simulink model "RateAdaptive"  (R2020a)
settings: Solver=FixedStepAuto  StartTime=0.0  StopTime=10.0  FixedStep=1e-3  RelTol=1e-3  EnableMultiTasking=on
settings Model: ExtModeTrigDuration=5  Creator=WinnieTrandinh  LastModifiedBy=WinnieTrandinh
settings OptimizationCC: EnhancedBackFolding=on  PassReuseOutputArgsAs=Individual arguments  ZeroExternalMemoryAtStartup=off  ZeroInternalMemoryAtStartup=off  MaxStackSize=64  OptimizeBlockOrder=speed  DifferentSizesBufferReuse=on  OptimizationCustomize=off  EfficientTunableParamExpr=on
settings DebuggingCC: ParameterTunabilityLossMsg=error
settings HardwareCC: ProdBitPerPointer=32  ProdBitPerSizeT=32  ProdBitPerPtrDiffT=32  ProdLargestAtomicInteger=Long  ProdLargestAtomicFloat=Double  ProdWordSize=32  ProdHWDeviceType=ARM Compatible->ARM Cortex
settings SFSimCC: MATLABDynamicMemAlloc=off
settings RTWCC: SystemTargetFile=ert.tlc  HardwareBoard=NXP FRDM-K64F  TemplateMakefile=ert_default_tmf  Toolchain=GNU Tools for ARM Embedded Processors
settings CodeAppCC: ForceParamTrailComments=on  IgnoreCustomStorageClasses=off  OperatorAnnotations=on  SimulinkDataObjDesc=on  SFDataObjDesc=on  InsertBlockDesc=on

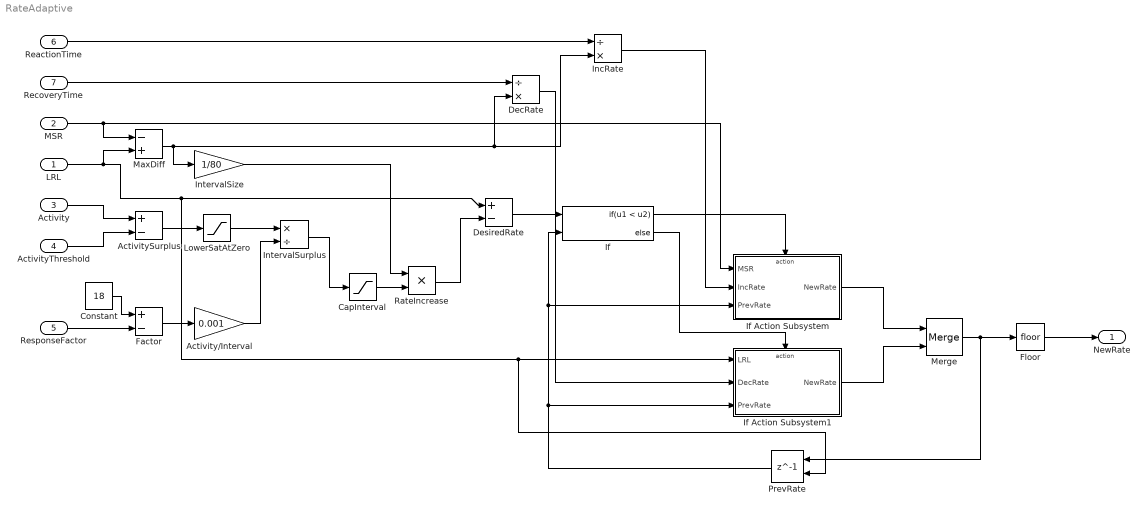
== system RateAdaptive ==
  LRL : Inport  Unit=ms
  MSR : Inport  Port=2  Unit=ms
  Activity : Inport  Port=3
  ActivityThreshold : Inport  Port=4
  ResponseFactor : Inport  Port=5
  ReactionTime : Inport  Port=6  Unit=ms
  RecoveryTime : Inport  Port=7  Unit=ms
  Activity/Interval : Gain  Gain=0.001
  ActivitySurplus : Sum  Inputs=+-
  CapInterval : Saturate  UpperLimit=80  LowerLimit=0
  Constant : Constant  Value=18
  DecRate : Product  Inputs=/*  OutDataTypeStr=double
  DesiredRate : Sum  Inputs=+-
  Factor : Sum  Inputs=+-
  Floor : Rounding
  If : If  NumInputs=2  IfExpression=u1 < u2
  If Action Subsystem : Subsystem  TreatAsAtomicUnit=on
  If Action Subsystem1 : Subsystem  TreatAsAtomicUnit=on
  IncRate : Product  Inputs=/*  OutDataTypeStr=double
  IntervalSize : Gain  Gain=1/80
  IntervalSurplus : Product  Inputs=*/
  LowerSatAtZero : Saturate  UpperLimit=inf  LowerLimit=0
  MaxDiff : Sum  Inputs=-+
  Merge : Merge
  PrevRate : Delay  DelayLength=1  InitialConditionSource=Input port
      settings: InputPortMap=u0,p4
  RateIncrease : Product  Inputs=**
  NewRate : Outport
  wires:
  CapInterval/1 -> RateIncrease/2
  Activity/Interval/1 -> IntervalSurplus/2
  IntervalSize/1 -> RateIncrease/1
  If/2 -> If Action Subsystem1/Action
  MaxDiff/1 -> IntervalSize/1, IncRate/2, DecRate/2
  Activity/1 -> ActivitySurplus/1
  If Action Subsystem/1(NewRate) -> Merge/1
  RecoveryTime/1 -> DecRate/1
  DecRate/1 -> If Action Subsystem1/2(DecRate)
  MSR/1 -> If Action Subsystem/1(MSR), MaxDiff/1
  Factor/1 -> Activity/Interval/1
  PrevRate/1 -> If/2, If Action Subsystem/3(PrevRate), If Action Subsystem1/3(PrevRate)
  LowerSatAtZero/1 -> IntervalSurplus/1
  Floor/1 -> NewRate/1
  ResponseFactor/1 -> Factor/2
  IncRate/1 -> If Action Subsystem/2(IncRate)
  Merge/1 -> Floor/1, PrevRate/1
  Constant/1 -> Factor/1
  If Action Subsystem1/1(NewRate) -> Merge/2
  RateIncrease/1 -> DesiredRate/2
  ReactionTime/1 -> IncRate/1
  If/1 -> If Action Subsystem/Action
  DesiredRate/1 -> If/1
  LRL/1 -> PrevRate/2, If Action Subsystem1/1(LRL), DesiredRate/1, MaxDiff/2
  IntervalSurplus/1 -> CapInterval/1
  ActivityThreshold/1 -> ActivitySurplus/2
  ActivitySurplus/1 -> LowerSatAtZero/1

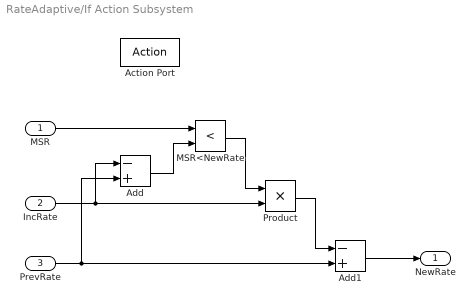
== system RateAdaptive/If Action Subsystem ==
  MSR : Inport
  IncRate : Inport  Port=2
  PrevRate : Inport  Port=3
  Action Port : ActionPort  ActionPortLabel=if(u1 < u2)
  Add : Sum  Inputs=-+
  Add1 : Sum  Inputs=-+
  MSR<NewRate : RelationalOperator  Operator=<  OutDataTypeStr=boolean  RndMeth=Simplest
  Product : Product
  NewRate : Outport
  wires:
  IncRate/1 -> Add/1, Product/2
  PrevRate/1 -> Add1/2, Add/2
  Add1/1 -> NewRate/1
  Product/1 -> Add1/1
  Add/1 -> MSR<NewRate/2
  MSR/1 -> MSR<NewRate/1
  MSR<NewRate/1 -> Product/1

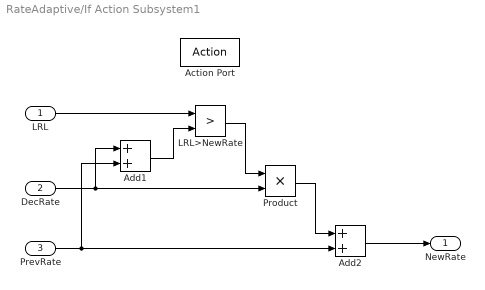
== system RateAdaptive/If Action Subsystem1 ==
  LRL : Inport
  DecRate : Inport  Port=2
  PrevRate : Inport  Port=3
  Action Port : ActionPort  ActionPortLabel=else
  Add1 : Sum
  Add2 : Sum
  LRL>NewRate : RelationalOperator  Operator=>  OutDataTypeStr=boolean  RndMeth=Simplest
  Product : Product
  NewRate : Outport
  wires:
  LRL/1 -> LRL>NewRate/1
  Add1/1 -> LRL>NewRate/2
  LRL>NewRate/1 -> Product/1
  Product/1 -> Add2/1
  PrevRate/1 -> Add2/2, Add1/2
  Add2/1 -> NewRate/1
  DecRate/1 -> Add1/1, Product/2
